simulink model "secordermodeldcmotorflywheel"  (R2025b)
settings: Solver=VariableStepAuto  StartTime=0.0  StopTime=10.0  RelTol=1e-3
settings Model: Creator=daryl  LastModifiedBy=daryl

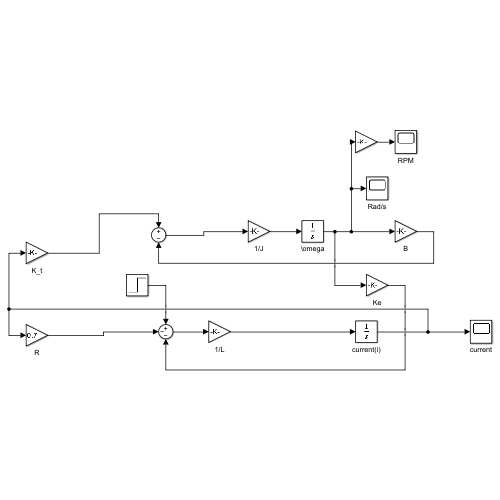
[thumbnail: Simulink's stored preview of the top-level diagram]
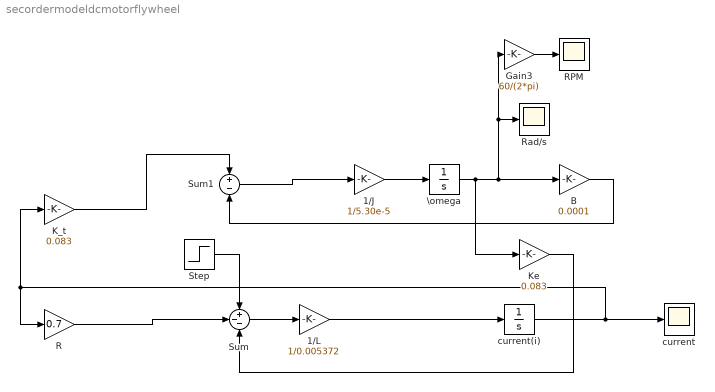
== system secordermodeldcmotorflywheel ==
  1/J : Gain  Gain=1/5.30e-5
  1/L : Gain  Gain=1/0.005372
  B : Gain  Gain=0.0001
  Gain3 : Gain  Gain=60/(2*pi)
  K_t : Gain  Gain=0.083
  Ke : Gain  Gain=0.083
  R : Gain  Gain=0.7
  RPM : Scope
      settings: ActiveDisplayYMinimum=-17373.017238077242  ActiveDisplayYMaximum=156357.15514269521
  Rad/s : Scope
      settings: ActiveDisplayYMinimum=-1819.2981108610763  ActiveDisplayYMaximum=16373.682997749691
  Step : Step  After=1000  SampleTime=0
  Sum : Sum  Inputs=+--
  Sum1 : Sum  Inputs=+-
  \omega : Integrator
  current : Scope
      settings: ActiveDisplayYMinimum=-250.44615091324852  ActiveDisplayYMaximum=814.58997883570464  DataLoggingVariableName=ScopeData2
  current(i) : Integrator
  wires:
  Step/1 -> Sum/1
  R/1 -> Sum/2
  Sum/1 -> 1/L/1
  K_t/1 -> Sum1/1
  Sum1/1 -> 1/J/1
  1/J/1 -> \omega/1
  B/1 -> Sum1/2
  Gain3/1 -> RPM/1
  1/L/1 -> current(i)/1
  current(i)/1 -> R/1, K_t/1, current/1
  \omega/1 -> Ke/1, Gain3/1, Rad/s/1, B/1
  Ke/1 -> Sum/3
